simulink model "Pokus15_Graphic_Display"  (Simulink 8.1)
settings: Solver=FixedStepDiscrete  StartTime=0.0  StopTime=10.0  RelTol=1e-3
libraries: Memory_Blocks_Lib x16, commutil2 x2, simulink_extras x1, Decoders_Lib x1, dspsnks4 x1
settings Model: Creator=uzivatel  LastModifiedBy=uzivatel
settings DataIOCC: SignalLoggingSaveFormat=Dataset
settings OptimizationCC: ExpressionDepthLimit=128
settings DebuggingCC: FcnCallInpInsideContextMsg=EnableAllAsError
settings GRTTargetCC: CombineOutputUpdateFcns=on  GRTInterface=off

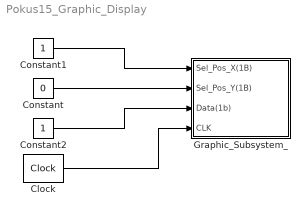
== system Pokus15_Graphic_Display ==
  Clock : simulink_extras/Flip Flops/Clock  period=2
  Constant : Constant  Value=0  OutDataTypeStr=uint8
  Constant1 : Constant  OutDataTypeStr=uint8
  Constant2 : Constant  OutDataTypeStr=boolean
  Graphic_Subsystem_ : Subsystem
  wires:
  Constant/1 -> Graphic_Subsystem_/2(Sel_Pos_Y(1B))
  Constant1/1 -> Graphic_Subsystem_/1(Sel_Pos_X(1B))
  Constant2/1 -> Graphic_Subsystem_/3(Data(1b))
  Clock/1 -> Graphic_Subsystem_/4(CLK)

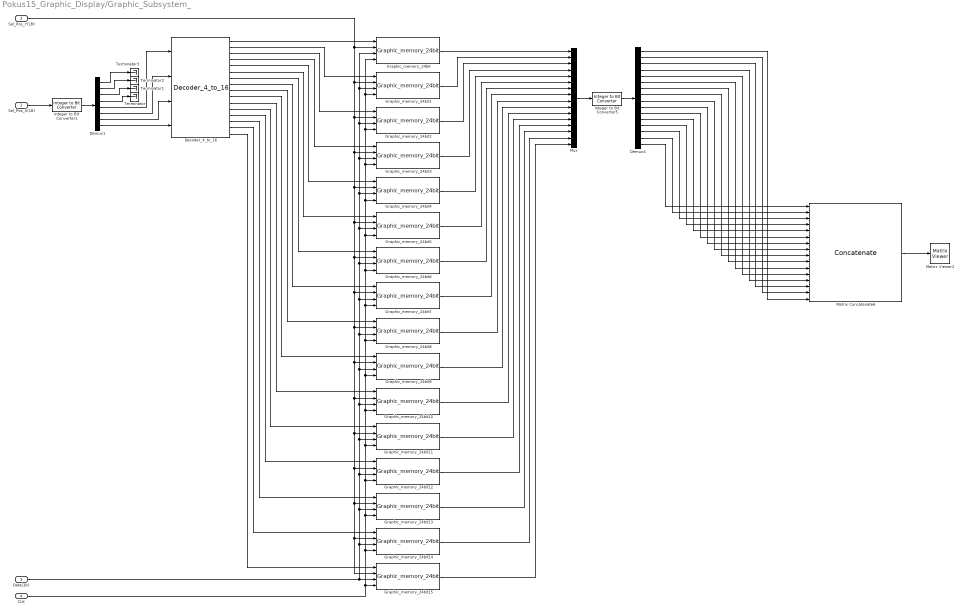
== system Pokus15_Graphic_Display/Graphic_Subsystem_ ==
  Sel_Pos_X(1B) : Inport
  Sel_Pos_Y(1B) : Inport  Port=2
  Data(1b) : Inport  Port=3
  CLK : Inport  Port=4
  Decoder_4_to_16 : Decoders_Lib/Decoders_Lib/Decoder_4_to_16
  Demux1 : Demux  Outputs=8
  Demux4 : Demux  Outputs=16
  Graphic_memory_24bit{,1..15} (16 alike) : Memory_Blocks_Lib/Memory_Blocks_Lib/Graphic_memory_24bit
  Integer to Bit Converter1 : commutil2/Integer to Bit Converter  nbits=8  signedInputValues=Unsigned  bitOrder=MSB first  outDtype=uint8
  Integer to Bit Converter5 : commutil2/Integer to Bit Converter  nbits=24  signedInputValues=Unsigned  bitOrder=LSB first  outDtype=uint32
  Matrix Concatenate6 : Concatenate  NumInputs=16  Mode=Multidimensional array  ConcatenateDimension=2
  Matrix Viewer2 : dspsnks4/Matrix Viewer  ImageParams=off  CMapStr=[0 0.3 0; 0 1 0]  AxisColorbar=on  AxisParams=off  AxisOrigin=Upper left corner  XLabel=X-axis  YLabel=Y-axis  ZLabel=Z-axis  FigPos=[1700 500 200 350]  AxisZoom=on
      settings: YMin=0  YMax=1
  Mux : Mux  Inputs=16
  Terminator{,1..3} (4 alike) : Terminator
  wires:
  Sel_Pos_Y(1B)/1 -> Graphic_memory_24bit1/2, Graphic_memory_24bit2/2, Graphic_memory_24bit3/2, Graphic_memory_24bit4/2, Graphic_memory_24bit5/2, Graphic_memory_24bit6/2, Graphic_memory_24bit7/2, Graphic_memory_24bit8/2, Graphic_memory_24bit9/2, Graphic_memory_24bit10/2, Graphic_memory_24bit11/2, Graphic_memory_24bit12/2, Graphic_memory_24bit13/2, Graphic_memory_24bit14/2, Graphic_memory_24bit15/2, Graphic_memory_24bit/2
  Demux1/1 -> Terminator3/1
  Demux1/2 -> Terminator2/1
  Demux1/5 -> Decoder_4_to_16/1
  Demux1/7 -> Decoder_4_to_16/3
  Sel_Pos_X(1B)/1 -> Integer to Bit Converter1/1
  Data(1b)/1 -> Graphic_memory_24bit14/3, Graphic_memory_24bit13/3, Graphic_memory_24bit12/3, Graphic_memory_24bit11/3, Graphic_memory_24bit10/3, Graphic_memory_24bit9/3, Graphic_memory_24bit8/3, Graphic_memory_24bit7/3, Graphic_memory_24bit6/3, Graphic_memory_24bit5/3, Graphic_memory_24bit4/3, Graphic_memory_24bit3/3, Graphic_memory_24bit2/3, Graphic_memory_24bit1/3, Graphic_memory_24bit/3, Graphic_memory_24bit15/3
  Demux1/6 -> Decoder_4_to_16/2
  Demux1/8 -> Decoder_4_to_16/4
  Integer to Bit Converter1/1 -> Demux1/1
  Demux1/4 -> Terminator/1
  Demux1/3 -> Terminator1/1
  Mux/1 -> Integer to Bit Converter5/1
  Decoder_4_to_16/13 -> Graphic_memory_24bit12/1
  Matrix Concatenate6/1 -> Matrix Viewer2/1
  Integer to Bit Converter5/1 -> Demux4/1
  Graphic_memory_24bit2/1 -> Mux/3
  Decoder_4_to_16/6 -> Graphic_memory_24bit5/1
  Graphic_memory_24bit9/1 -> Mux/10
  Decoder_4_to_16/11 -> Graphic_memory_24bit10/1
  Graphic_memory_24bit4/1 -> Mux/5
  Graphic_memory_24bit/1 -> Mux/1
  Graphic_memory_24bit13/1 -> Mux/14
  Decoder_4_to_16/3 -> Graphic_memory_24bit2/1
  Graphic_memory_24bit15/1 -> Mux/16
  Decoder_4_to_16/16 -> Graphic_memory_24bit15/1
  CLK/1 -> Graphic_memory_24bit14/4, Graphic_memory_24bit13/4, Graphic_memory_24bit12/4, Graphic_memory_24bit11/4, Graphic_memory_24bit10/4, Graphic_memory_24bit9/4, Graphic_memory_24bit8/4, Graphic_memory_24bit7/4, Graphic_memory_24bit6/4, Graphic_memory_24bit5/4, Graphic_memory_24bit4/4, Graphic_memory_24bit3/4, Graphic_memory_24bit2/4, Graphic_memory_24bit1/4, Graphic_memory_24bit/4, Graphic_memory_24bit15/4
  Decoder_4_to_16/1 -> Graphic_memory_24bit/1
  Graphic_memory_24bit3/1 -> Mux/4
  Decoder_4_to_16/10 -> Graphic_memory_24bit9/1
  Graphic_memory_24bit12/1 -> Mux/13
  Decoder_4_to_16/12 -> Graphic_memory_24bit11/1
  Graphic_memory_24bit5/1 -> Mux/6
  Graphic_memory_24bit1/1 -> Mux/2
  Decoder_4_to_16/2 -> Graphic_memory_24bit1/1
  Decoder_4_to_16/4 -> Graphic_memory_24bit3/1
  Decoder_4_to_16/9 -> Graphic_memory_24bit8/1
  Graphic_memory_24bit11/1 -> Mux/12
  Decoder_4_to_16/5 -> Graphic_memory_24bit4/1
  Graphic_memory_24bit6/1 -> Mux/7
  Graphic_memory_24bit7/1 -> Mux/8
  Graphic_memory_24bit8/1 -> Mux/9
  Decoder_4_to_16/14 -> Graphic_memory_24bit13/1
  Graphic_memory_24bit14/1 -> Mux/15
  Decoder_4_to_16/15 -> Graphic_memory_24bit14/1
  Decoder_4_to_16/8 -> Graphic_memory_24bit7/1
  Decoder_4_to_16/7 -> Graphic_memory_24bit6/1
  Graphic_memory_24bit10/1 -> Mux/11
  Demux4/16 -> Matrix Concatenate6/1
  Demux4/15 -> Matrix Concatenate6/2
  Demux4/14 -> Matrix Concatenate6/3
  Demux4/13 -> Matrix Concatenate6/4
  Demux4/12 -> Matrix Concatenate6/5
  Demux4/11 -> Matrix Concatenate6/6
  Demux4/10 -> Matrix Concatenate6/7
  Demux4/9 -> Matrix Concatenate6/8
  Demux4/8 -> Matrix Concatenate6/9
  Demux4/7 -> Matrix Concatenate6/10
  Demux4/6 -> Matrix Concatenate6/11
  Demux4/5 -> Matrix Concatenate6/12
  Demux4/4 -> Matrix Concatenate6/13
  Demux4/3 -> Matrix Concatenate6/14
  Demux4/2 -> Matrix Concatenate6/15
  Demux4/1 -> Matrix Concatenate6/16
